simulink model "Semi_Final_integration"  (R2023b)
settings: Solver=FixedStepAuto  StartTime=0.0  StopTime=inf  FixedStep=Ts  RelTol=1e-3
InitFcn:
  | params
  | pin_params
values from neighbouring files (symbols this model uses):
  b = 100    [params.m]
  default1 = 360    [params.m]
  den_Gd = Gd.Den{:}    [params.m]
  encoder_scale = 1/12/4 *2*pi    (= 0.1308996939)    [params.m]
  f = 100    [params.m]
  J = 0.02    [params.m]
  Kb = 0.1    [params.m]
  KD = 0    [params.m]
  Kf = 0.01    [params.m]
  KI = 0.03    [params.m]
  Km = 1    [params.m]
  KP = 0.009    [params.m]
  l = 100    [params.m]
  L = 0.5    [params.m]
  num_Gd = Gd.Num{:}    [params.m]
  r = 100    [params.m]
  R = 2.0    (= 2)    [params.m]
  steering = 0.02    [params.m]
  Vlim = 12    [params.m]
undefined symbols (not defined in the file or in its folder): Wref
libraries: arduinolib x29, arduinosensorlib x17, simulink x6
(part 1 of 2)
settings Model: SimulationMode=external  ExtModeTrigDuration=2  Creator=SJ  LastModifiedBy=SJ
settings SolverCC: AutoInsertRateTranBlk=on
settings OptimizationCC: EnhancedBackFolding=on  PassReuseOutputArgsAs=Individual arguments  ZeroExternalMemoryAtStartup=off  ZeroInternalMemoryAtStartup=off  MaxStackSize=64  OptimizeBlockOrder=speed  DifferentSizesBufferReuse=on  OptimizationCustomize=off  EfficientTunableParamExpr=on
settings DebuggingCC: MultiTaskRateTransMsg=warning  ParameterTunabilityLossMsg=error
settings HardwareCC: ProdBitPerInt=16  ProdBitPerPointer=16  ProdBitPerSizeT=16  ProdBitPerPtrDiffT=16  ProdLargestAtomicFloat=None  ProdWordSize=8  ProdHWDeviceType=Atmel->AVR
settings SFSimCC: MATLABDynamicMemAlloc=off
settings RTWCC: Description=Embedded Coder  SystemTargetFile=ert.tlc  HardwareBoard=Arduino Mega 2560  TemplateMakefile=ert_default_tmf  Toolchain=Arduino AVR  BuildConfiguration=Faster Runs
settings CodeAppCC: ForceParamTrailComments=on  IgnoreCustomStorageClasses=off  OperatorAnnotations=on  SimulinkDataObjDesc=on  SFDataObjDesc=on  InsertBlockDesc=on
settings ERTTargetCC: SupportContinuousTime=on  SupportVariableSizeSignals=on  ExtMode=on  ExtModeTransport=3  ExtModeStaticAlloc=on  ExtModeAutomaticAllocSize=off  ExtModeStaticAllocSize=2048  ExtModeMexFile=ext_xcp  ExtModeMexArgs=0 13 921600  ExtModeIntrfLevel=Level2 - Open

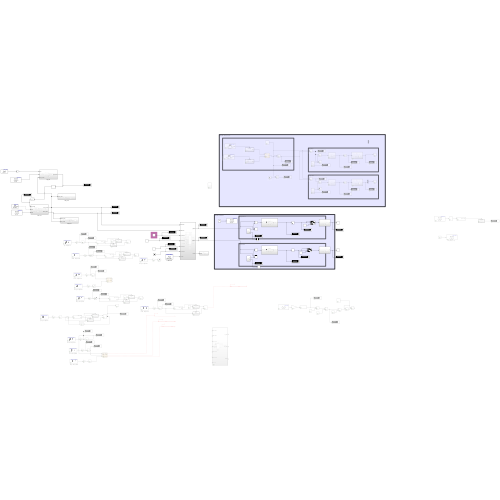
[thumbnail: Simulink's stored preview of the top-level diagram]
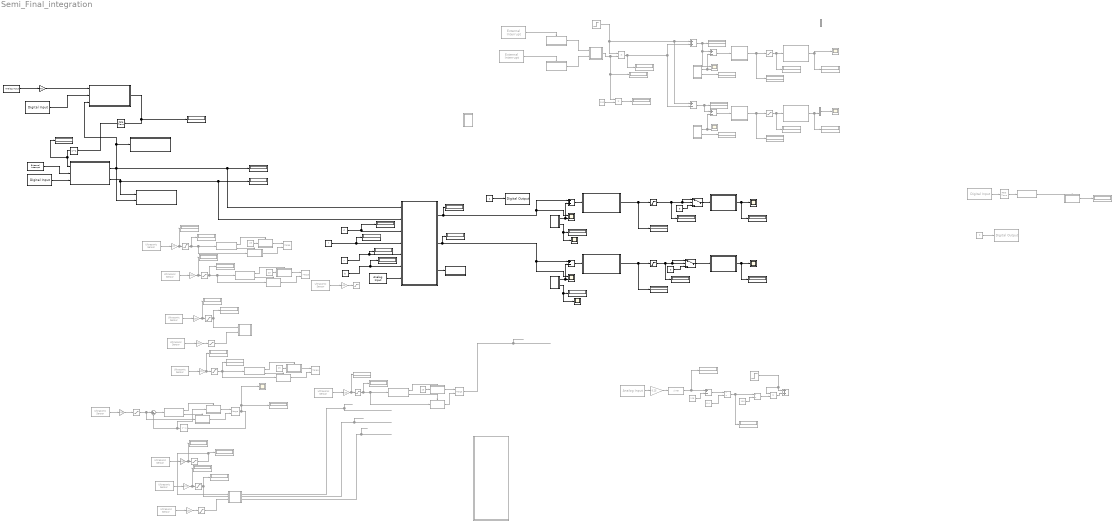
== system Semi_Final_integration ==
  note: Subsystem3
  note: Subsystem13
  note: Left Motor
  note: Variable resistance
  note: sw1,2로 1퍼 증가, 감소
  note: Right Motor
  Add : Sum  Commented=on
  Add{1..2,7..8} (4 alike) : Sum  Commented=on  Inputs=+-
  Add3 : Sum
  Add4 : Sum  Commented=on
  Add5 : Sum  Inputs=+-
  Analog Input : arduinolib/Analog Input  Commented=on  pinNumber=8  ReadResultsOnly=off  ConversionTriggerSource=Software  ExternalTriggerType=uint32( 0 )  OutputDataType=uint16  EnableConversionCompleteNotify=off  EnableOuputStatus=off  SampleTime=-1  blockPlatform=arduino
  Analog Input1 : arduinolib/Analog Input  pinNumber=BS  ReadResultsOnly=off  ConversionTriggerSource=Software  ExternalTriggerType=uint32( 0 )  OutputDataType=uint16  EnableConversionCompleteNotify=off  EnableOuputStatus=off  SampleTime=-1  blockPlatform=arduino
  Chart : Stateflow chart  Commented=on  TreatAsAtomicUnit=on
  Chart1 : Stateflow chart  Commented=on  TreatAsAtomicUnit=on
      settings: PortSchema="{\"entries\":[{\"content\":{\"sides\":[{\"content\":{\"connectorIds\":[\"In1\",\"In2\"]},\"type\":\"ConnectorPlacement.EquallySpacedRectSide\",\"uuid\":\"caf7ae87-23bd-4c3e-9883-bf517c2acc71\"},{\"content\":{\"connectorIds\":[\"Out2\",\"Out1\"],\"side\":\"RIGHT\"},\"type\":\"ConnectorPlacement.EquallySpacedRectSide\",\"uuid\":\"5b72cbb9-a353-4fa8-8bce-0f613714d9b8\"},{\"content\":{\"side\":\"TOP\"},\"type\":\"ConnectorPlacement.EquallySpacedRectSide\",\"uuid\":\"2518c824-60ae-4861-9582-6b6ed29bfb4f\"}]},\"type\":\"ConnectorPlacement.EquallySpacedConnector\",\"uuid\":\"4f310b78-9bfc-4c18-9eab-8f3bf0529cab\"}],\"packageUris\":[\"http://schema.mathworks.com/mf0/Connector/R2020b\"],\"version\":\"1.0\"}"
  Chart2 : Stateflow chart  Commented=on  TreatAsAtomicUnit=on
      settings: PortSchema="{\"entries\":[{\"content\":{\"sides\":[{\"content\":{\"connectorIds\":[\"In1\",\"In2\",\"In3\"]},\"type\":\"ConnectorPlacement.EquallySpacedRectSide\",\"uuid\":\"caf7ae87-23bd-4c3e-9883-bf517c2acc71\"},{\"content\":{\"connectorIds\":[\"Out1\",\"Out3\",\"Out2\"],\"side\":\"RIGHT\"},\"type\":\"ConnectorPlacement.EquallySpacedRectSide\",\"uuid\":\"5b72cbb9-a353-4fa8-8bce-0f613714d9b8\"},{\"content\":{\"side\":\"TOP\"},\"type\":\"ConnectorPlacement.EquallySpacedRectSide\",\"uuid\":\"2518c824-60ae-4861-9582-6b6ed29bfb4f\"}]},\"type\":\"ConnectorPlacement.EquallySpacedConnector\",\"uuid\":\"4f310b78-9bfc-4c18-9eab-8f3bf0529cab\"}],\"packageUris\":[\"http://schema.mathworks.com/mf0/Connector/R2020b\"],\"version\":\"1.0\"}"
  Constant : Constant  Commented=on  Value=128
  Constant1 : Constant  Commented=on  Value=6.4
  Constant{10..12,15} (4 alike) : Constant  Commented=on  Value=25
  Constant13 : Constant
  Constant16 : Constant  Value=0
  Constant2 : Constant  Commented=on  Value=100
  Constant3 : Constant  Commented=on  Value=100
  Constant4 : Constant  Value=f
  Constant5 : Constant  Commented=on  Value=0
  Constant6 : Constant  Value=l
  Constant7 : Constant  Value=b
  Constant8 : Constant  Value=r
  Constant9 : Constant  Value=0
  Data Type Conversion : DataTypeConversion  Commented=on  OutDataTypeStr=uint8  SaturateOnIntegerOverflow=off  RndMeth=Floor
  Delay : Delay  DelayLength=1
  Delay1 : Delay  Commented=on  DelayLength=1
  Digital Input : arduinolib/Digital Input  Commented=on  pinNumber=20  mode=Default  Direction=input  SampleTime=0.1  blockPlatform=arduino
  Digital Input1 : arduinolib/Digital Input  pinNumber=SW3  mode=Default  Direction=input  SampleTime=0.1  blockPlatform=arduino
  Digital Input2 : arduinolib/Digital Input  pinNumber=SW2  mode=Default  Direction=input  SampleTime=0.1  blockPlatform=arduino
  Digital Output : arduinolib/Digital Output  pinNumber=13  Direction=output  blockPlatform=arduino
  Display{,1..7,12,17..23,34..44,47..50} (31 alike) : Display  Commented=on
  Display{8..11,13..16,24..33} (18 alike) : Display
  Divide : Product  Commented=on  Inputs=**
  Divide1 : Product  Commented=on  Inputs=*/
  Divide2 : Product  Commented=on  Inputs=**
  Divide3 : Product  Commented=on  Inputs=*/
  Divide4 : Product  Commented=on  Inputs=**
  External Interrupt : arduinolib/External Interrupt  Commented=on  Pin=20  PullUp=off  Mode=FALLING  InterruptSimulationInput=off
  External Interrupt1 : arduinolib/External Interrupt  Commented=on  Pin=21  PullUp=off  Mode=FALLING  InterruptSimulationInput=off
  External Interrupt2 : arduinolib/External Interrupt  Pin=SW1  PullUp=off  Mode=RISING  InterruptSimulationInput=off
  Function-Call Subsystem1 : Subsystem  Commented=on  TreatAsAtomicUnit=on
  Function-Call Subsystem4 : Subsystem  Commented=on  TreatAsAtomicUnit=on
  Gain : Gain  Commented=on  Gain=0.25
  Gain{1..11} (11 alike) : Gain  Commented=on  Gain=100
  Gain12 : Gain  Gain=70
  If : If  Commented=on  IfExpression=u1 == 0  ShowElse=off
  If Action Subsystem : Subsystem  Commented=on  TreatAsAtomicUnit=on
  If Action Subsystem1 : Subsystem  Commented=on  TreatAsAtomicUnit=on
  If Action Subsystem10 : Subsystem  Commented=on  TreatAsAtomicUnit=on
  If Action Subsystem11 : Subsystem  Commented=on  TreatAsAtomicUnit=on
  If Action Subsystem12 : Subsystem  Commented=on  TreatAsAtomicUnit=on
  If Action Subsystem2 : Subsystem  Commented=on  TreatAsAtomicUnit=on
  If Action Subsystem3 : Subsystem  Commented=on  TreatAsAtomicUnit=on
  If Action Subsystem4 : Subsystem  Commented=on  TreatAsAtomicUnit=on
  If Action Subsystem5 : Subsystem  Commented=on  TreatAsAtomicUnit=on
  If Action Subsystem6 : Subsystem  Commented=on  TreatAsAtomicUnit=on
  If Action Subsystem7 : Subsystem  Commented=on  TreatAsAtomicUnit=on
  If1 : If  Commented=on  IfExpression=u1 > 25
  If2 : If  Commented=on  IfExpression=u1 > 12
  If3 : If  Commented=on  IfExpression=u1 > 25
  If5 : If  Commented=on  IfExpression=u1 > 12
  If6 : If  Commented=on  IfExpression=u1 > 25
  LED_B Ctrl : Subsystem
  LED_R Ctrl : Subsystem
  Merge{1..3,5..6} (5 alike) : Merge  Commented=on
  Mux1 : Mux  Commented=on  Inputs=2
  Mux4 : Mux  Commented=on  Inputs=2
  R_Motor(반시계) : arduinolib/Digital Output  Commented=on  pinNumber=Motor_R_Direction  Direction=output  blockPlatform=arduino
  Rate Transition : RateTransition  Commented=on  OutPortSampleTime=0.5
  Rate Transition1 : RateTransition  Integrity=off
  Saturation : Saturate  Commented=on  UpperLimit=12  LowerLimit=0
  Saturation1 : Saturate  UpperLimit=12  LowerLimit=2
  Saturation{4..6,9..11,13..14} (8 alike) : Saturate  Commented=on  UpperLimit=30  LowerLimit=0
  Saturation12 : Saturate  Commented=on  UpperLimit=15  LowerLimit=0
  Saturation2 : Saturate  UpperLimit=12  LowerLimit=0
  Saturation3 : Saturate  Commented=on  UpperLimit=12  LowerLimit=0
  Saturation7 : Saturate  Commented=on  UpperLimit=15  LowerLimit=0
  Saturation8 : Saturate  Commented=on  UpperLimit=15  LowerLimit=0
  Scope : Scope  Commented=on  NumInputPorts=2
  Scope1 : Scope  NumInputPorts=2
  Scope{2,5,9..10} (4 alike) : Scope
  Scope3 : Scope  Commented=on
  Scope4 : Scope  NumInputPorts=2
  Scope6 : Scope  Commented=on  NumInputPorts=2
  Scope7 : Scope  Commented=on
  Scope8 : Scope  Commented=on
  State_Ctrl : Subsystem
  Step : Step  Commented=on  After=Wref  SampleTime=0
  Step1 : Step  Commented=on  After=Wref  SampleTime=0
  Subsystem : Subsystem  Commented=on
  Subsystem1 : Subsystem  Commented=on
  Subsystem10 : Subsystem  Commented=on
  Subsystem11 : Subsystem  Commented=on
  Subsystem12 : Subsystem  Commented=on
  Subsystem13 : Subsystem
  Subsystem14 : Subsystem
  Subsystem15 : Subsystem
  Subsystem2 : Subsystem  Commented=on
  Subsystem3 : Subsystem
  Subsystem4 : Subsystem
  Subsystem5 : Subsystem  Commented=on
  Subsystem6 : Subsystem  Commented=on
  Subsystem7 : Subsystem
  Subsystem8 : Subsystem
  Subsystem9 : Subsystem
  Sum : Sum  Commented=on  Inputs=|+-
  Switch : Switch  Criteria=u2 > Threshold  Threshold=1.6  SaturateOnIntegerOverflow=off  InputSameDT=off
  Switch1 : Switch  Criteria=u2 > Threshold  Threshold=1.6  SaturateOnIntegerOverflow=off  InputSameDT=off
  light_Ctrl : Subsystem
  가변저항 : arduinolib/Analog Input  pinNumber=8  ReadResultsOnly=off  ConversionTriggerSource=Software  ExternalTriggerType=uint32( 0 )  OutputDataType=uint16  EnableConversionCompleteNotify=off  EnableOuputStatus=off  SampleTime=-1  blockPlatform=arduino
  앞 초음파1 : arduinosensorlib/Ultrasonic Sensor  Commented=on  NumSignalPins=2  TrigPin=F_Triger  EchoPin=F_Echo  SignalPin=3  SampleTime_=0.01  blockPlatform=ARDUINO
  우측 초음파1 : arduinosensorlib/Ultrasonic Sensor  Commented=on  NumSignalPins=2  TrigPin=R_Triger  EchoPin=R_Echo  SignalPin=3  SampleTime_=0.01  blockPlatform=ARDUINO
  우측 초음파2 : arduinosensorlib/Ultrasonic Sensor  Commented=on  NumSignalPins=2  TrigPin=R_Triger  EchoPin=R_Echo  SignalPin=3  SampleTime_=0.01  blockPlatform=ARDUINO
  우측 초음파3 : arduinosensorlib/Ultrasonic Sensor  Commented=on  NumSignalPins=2  TrigPin=R_Triger  EchoPin=R_Echo  SignalPin=3  SampleTime_=0.01  blockPlatform=ARDUINO
  전방 초음파1 : arduinosensorlib/Ultrasonic Sensor  Commented=on  NumSignalPins=2  TrigPin=F_Triger  EchoPin=F_Echo  SignalPin=3  SampleTime_=0.01  blockPlatform=ARDUINO
  좌측 초음파2 : arduinosensorlib/Ultrasonic Sensor  Commented=on  NumSignalPins=2  TrigPin=L_Triger  EchoPin=L_Echo  SignalPin=3  SampleTime_=0.01  blockPlatform=ARDUINO
  좌측 초음파3 : arduinosensorlib/Ultrasonic Sensor  Commented=on  NumSignalPins=2  TrigPin=L_Triger  EchoPin=L_Echo  SignalPin=3  SampleTime_=0.01  blockPlatform=ARDUINO
  후방 초음파{1..4} (4 alike) : arduinosensorlib/Ultrasonic Sensor  Commented=on  NumSignalPins=2  TrigPin=B_Triger  EchoPin=B_Echo  SignalPin=3  SampleTime_=0.01  blockPlatform=ARDUINO
  wires:
  Subsystem/1(Out1) -> Add1/2, Scope/2
  Saturation/1 -> Subsystem1/1(In2), Display/1
  Subsystem1/1(Out1) -> Scope3/1, Display3/1
  External Interrupt/1 -> Function-Call Subsystem4/Trigger
  External Interrupt1/1 -> Function-Call Subsystem1/Trigger
  Function-Call Subsystem4/1(sw1) -> Chart/1(sw1)
  Function-Call Subsystem1/1(sw2) -> Chart/2(sw2)
  Step/1 -> Divide/1, Add8/1, Add/1
  Divide/1 -> Display1/1, Add/2, Add8/2
  Chart/1(n) -> Divide4/1, Display7/1, Divide/2
  Subsystem/2(Out2) -> Display5/1
  Add/1 -> Scope/1, Add1/1, Display4/1
  Subsystem6/1(Out1) -> Display2/1, Saturation/1
  Add1/1 -> Subsystem6/1(In1)
  Add7/1 -> Subsystem12/1(In1)
  Subsystem11/1(Out1) -> Display19/1, Mux4/2
  Saturation3/1 -> Subsystem11/1(In2), Display17/1
  Mux4/1 -> Scope7/1
  Subsystem10/1(Out1) -> Add7/2, Scope6/2
  Subsystem12/1(Out1) -> Display18/1, Saturation3/1
  Subsystem10/2(Out2) -> Display20/1
  Add8/1 -> Add7/1, Display21/1
  Divide4/1 -> Display22/1
  Constant3/1 -> Divide4/2
  Digital Input/1 -> Rate Transition/1
  If/1 -> If Action Subsystem/Action
  If Action Subsystem/1(Out1) -> Display23/1
  Rate Transition/1 -> If/1
  Constant5/1 -> R_Motor(반시계)/1
  Digital Input1/1 -> light_Ctrl/2(In2)
  light_Ctrl/1(light_mode) -> Display10/1, Rate Transition1/1
  Analog Input1/1 -> Gain12/1
  Rate Transition1/1 -> Delay/1
  External Interrupt2/1 -> State_Ctrl/2(SW1)
  Delay/1 -> Display11/1, State_Ctrl/1(light_mode)
  Digital Input2/1 -> State_Ctrl/3(SW2)
  Add2/1 -> Divide1/1
  Data Type Conversion/1 -> Display12/1, Add2/1
  Gain/1 -> Data Type Conversion/1
  Constant/1 -> Add2/2
  Constant2/1 -> Divide3/2
  Step1/1 -> Add4/1, Divide2/1
  Divide3/1 -> Divide2/2
  Constant1/1 -> Divide1/2
  Analog Input/1 -> Gain/1
  Divide2/1 -> Add4/2
  Divide1/1 -> Display6/1, Divide3/1
  가변저항/1 -> Subsystem4/7(가변저항)
  Subsystem4/1(L_Motor) -> Add3/1, Scope1/1, Display24/1
  Subsystem8/1(Out1) -> Scope2/1, Display26/1
  Subsystem7/1(Out1) -> Add3/2, Scope1/2
  Subsystem9/1(Out1) -> Display29/1, Saturation1/1
  Subsystem7/2(Out2) -> Scope10/1, Display27/1
  Add3/1 -> Subsystem9/1(In1)
  Subsystem4/2(R_Motor) -> Scope4/1, Add5/1, Display25/1
  Subsystem14/1(Out1) -> Scope5/1, Display30/1
  Subsystem13/1(Out1) -> Add5/2, Scope4/2
  Subsystem15/1(Out1) -> Display33/1, Saturation2/1
  Subsystem13/2(Out2) -> Scope9/1, Display31/1
  Add5/1 -> Subsystem15/1(In1)
  우측 초음파2/1 -> Gain3/1
  Gain3/1 -> Display35/1, Saturation4/1
  Saturation4/1 -> Chart1/1(RUS), Display34/1
  Delay1/1 -> If Action Subsystem6/1(In1), Sum/2
  전방 초음파1/1 -> Gain2/1
  Sum/1 -> If3/1
  Merge3/1 -> Scope8/1, Display36/1, Delay1/1
  If Action Subsystem7/1(전방 초음파) -> Merge3/2
  If3/2 -> If Action Subsystem7/Action
  Gain2/1 -> Saturation5/1
  Saturation5/1 -> If Action Subsystem7/1(In1), Sum/1
  If Action Subsystem6/1(Out1) -> Merge3/1
  If3/1 -> If Action Subsystem6/Action
  Constant10/1 -> If Action Subsystem1/1(In1)
  If Action Subsystem2/1(전방 초음파) -> Merge1/2
  Saturation6/1 -> If1/1, Display37/1, If Action Subsystem2/1(In1)
  If1/2 -> If Action Subsystem2/Action
  Gain1/1 -> Display38/1, Saturation6/1
  If1/1 -> If Action Subsystem1/Action
  후방 초음파1/1 -> Gain1/1
  If Action Subsystem1/1(Out1) -> Merge1/1
  좌측 초음파2/1 -> Gain4/1
  If Action Subsystem3/1(Out1) -> Merge2/1
  If2/1 -> If Action Subsystem3/Action
  Gain4/1 -> Display40/1, Saturation7/1
  If2/2 -> If Action Subsystem4/Action
  If Action Subsystem4/1(전방 초음파) -> Merge2/2
  Constant11/1 -> If Action Subsystem3/1(In1)
  Saturation7/1 -> Display39/1, If2/1, If Action Subsystem4/1(In1)
  Saturation8/1 -> Display41/1, If5/1, If Action Subsystem10/1(In1)
  If5/1 -> If Action Subsystem5/Action
  앞 초음파1/1 -> Gain5/1
  If5/2 -> If Action Subsystem10/Action
  If Action Subsystem10/1(전방 초음파) -> Merge5/2
  If Action Subsystem5/1(Out1) -> Merge5/1
  Constant12/1 -> If Action Subsystem5/1(In1)
  Gain5/1 -> Display42/1, Saturation8/1
  State_Ctrl/1(Drive_mode) -> Subsystem4/1(drive mode), Display8/1, light_Ctrl/3(Drive_mode1), LED_R Ctrl/1(Drive_mode), LED_B Ctrl/2(Drive_mode)
  Constant4/1 -> Display16/1, Subsystem4/3(전방 초음파)
  Gain6/1 -> Saturation9/1
  후방 초음파2/1 -> Gain6/1
  Merge6/1 -> ?
  Constant15/1 -> If Action Subsystem11/1(In1)
  If Action Subsystem12/1(전방 초음파) -> Merge6/2
  Saturation10/1 -> Display43/1, If6/1, If Action Subsystem12/1(In1)
  If6/2 -> If Action Subsystem12/Action
  Gain7/1 -> Display44/1, Saturation10/1
  If6/1 -> If Action Subsystem11/Action
  우측 초음파1/1 -> Gain7/1
  If Action Subsystem11/1(Out1) -> Merge6/1
  Saturation9/1 -> Chart1/2(BUS)
  Gain11/1 -> Display50/1, Saturation12/1
  Gain10/1 -> Saturation14/1
  Chart2/2(data3) -> ?
  후방 초음파3/1 -> Gain10/1
  Chart2/1(data1) -> ?
  좌측 초음파3/1 -> Gain11/1
  Chart2/3(data2) -> ?
  Saturation14/1 -> Chart2/3(BUS)
  Gain9/1 -> Display48/1, Saturation13/1
  Saturation12/1 -> Display49/1, Chart2/1(LUS)
  Saturation13/1 -> Chart2/2(RUS), Display47/1
  우측 초음파3/1 -> Gain9/1
  Constant6/1 -> Display15/1, Subsystem4/4(좌측 초음파)
  Constant8/1 -> Display14/1, Subsystem4/5(우측 초음파)
  Gain8/1 -> Saturation11/1
  후방 초음파4/1 -> Gain8/1
  Subsystem4/3(buzzer) -> Subsystem3/1(buzzer)
  Constant7/1 -> Display13/1, Subsystem4/6(후방 초음파)
  Gain12/1 -> light_Ctrl/1(light1)
  Constant13/1 -> Digital Output/1
  State_Ctrl/2(ADAS_state1) -> LED_B Ctrl/1(ADAS_state), Subsystem4/2(adas mode), Display9/1
  Constant9/1 -> Switch/3
  Saturation2/1 -> Display28/1, Switch/1, Switch/2
  Switch/1 -> Subsystem14/1(In2)
  Saturation1/1 -> Switch1/1, Switch1/2, Display32/1
  Constant16/1 -> Switch1/3
  Switch1/1 -> Subsystem8/1(In2)

== system Semi_Final_integration/Function-Call Subsystem1 ==
  function : TriggerPort  TriggerType=function-call  VariantControl=(inherit)
  Add : Sum  Inputs=+-
  Constant : Constant
  Delay : Delay  DelayLength=1
  sw2 : Outport
  wires:
  Add/1 -> Delay/1, sw2/1
  Delay/1 -> Add/2
  Constant/1 -> Add/1

== system Semi_Final_integration/Function-Call Subsystem4 ==
  function : TriggerPort  TriggerType=function-call  VariantControl=(inherit)
  Add : Sum  Inputs=+-
  Constant : Constant
  Delay : Delay  DelayLength=1
  sw1 : Outport
  wires:
  Add/1 -> sw1/1, Delay/1
  Delay/1 -> Add/2
  Constant/1 -> Add/1

== system Semi_Final_integration/If Action Subsystem ==
  Action Port : ActionPort  ActionPortLabel=if(u1 == 0)
  Add : Sum
  Constant : Constant
  Constant1 : Constant  Value=3
  Delay : Delay  DelayLength=1
  Mod : Math  Operator=mod
  Out1 : Outport
  wires:
  Mod/1 -> Delay/1, Out1/1
  Delay/1 -> Add/2
  Constant/1 -> Add/1
  Add/1 -> Mod/1
  Constant1/1 -> Mod/2

== system Semi_Final_integration/If Action Subsystem1 ==
  In1 : Inport
  Action Port : ActionPort  ActionPortLabel=if(u1 > 25)
  Out1 : Outport
  wires:
  In1/1 -> Out1/1

== system Semi_Final_integration/If Action Subsystem10 ==
  In1 : Inport
  Action Port : ActionPort  ActionPortLabel=else
  전방 초음파 : Outport
  wires:
  In1/1 -> 전방 초음파/1

== system Semi_Final_integration/If Action Subsystem11 ==
  In1 : Inport
  Action Port : ActionPort  ActionPortLabel=if(u1 > 25)
  Out1 : Outport
  wires:
  In1/1 -> Out1/1

== system Semi_Final_integration/If Action Subsystem12 ==
  In1 : Inport
  Action Port : ActionPort  ActionPortLabel=else
  전방 초음파 : Outport
  wires:
  In1/1 -> 전방 초음파/1

== system Semi_Final_integration/If Action Subsystem2 ==
  In1 : Inport
  Action Port : ActionPort  ActionPortLabel=else
  전방 초음파 : Outport
  wires:
  In1/1 -> 전방 초음파/1

== system Semi_Final_integration/If Action Subsystem3 ==
  In1 : Inport
  Action Port : ActionPort  ActionPortLabel=if(u1 > 12)
  Out1 : Outport
  wires:
  In1/1 -> Out1/1

== system Semi_Final_integration/If Action Subsystem4 ==
  In1 : Inport
  Action Port : ActionPort  ActionPortLabel=else
  전방 초음파 : Outport
  wires:
  In1/1 -> 전방 초음파/1

== system Semi_Final_integration/If Action Subsystem5 ==
  In1 : Inport
  Action Port : ActionPort  ActionPortLabel=if(u1 > 12)
  Out1 : Outport
  wires:
  In1/1 -> Out1/1

== system Semi_Final_integration/If Action Subsystem6 ==
  In1 : Inport
  Action Port : ActionPort  ActionPortLabel=if(u1 > 25)
  Out1 : Outport
  wires:
  In1/1 -> Out1/1

== system Semi_Final_integration/If Action Subsystem7 ==
  In1 : Inport
  Action Port : ActionPort  ActionPortLabel=else
  전방 초음파 : Outport
  wires:
  In1/1 -> 전방 초음파/1

== system Semi_Final_integration/LED_B Ctrl ==
  ADAS_state : Inport
  Drive_mode : Inport  Port=2
  Constant : Constant
  Digital Output : arduinolib/Digital Output  pinNumber=LED1_B  Direction=output  blockPlatform=arduino
  If Action Subsystem1 : Subsystem  TreatAsAtomicUnit=on
  If Action Subsystem3 : Subsystem  TreatAsAtomicUnit=on
  If1 : If  IfExpression=u1 ==1
  Merge : Merge
  Product : Product
  Product1 : Product
  Pulse Generator : DiscretePulseGenerator  PulseType=Time based  PulseWidth=50
  wires:
  If1/2 -> If Action Subsystem3/Action
  If Action Subsystem1/1(Out1) -> Merge/1
  ADAS_state/1 -> If1/1
  If1/1 -> If Action Subsystem1/Action
  Merge/1 -> Digital Output/1
  If Action Subsystem3/1(Out1) -> Merge/2
  Drive_mode/1 -> Product/1, Product1/2
  Pulse Generator/1 -> Product/2
  Constant/1 -> Product1/1
  Product1/1 -> If Action Subsystem1/1(Input)
  Product/1 -> If Action Subsystem3/1(Input)

== system Semi_Final_integration/LED_R Ctrl ==
  Drive_mode : Inport
  Digital Output : arduinolib/Digital Output  pinNumber=LED1_R  Direction=output  blockPlatform=arduino
  If Action Subsystem1 : Subsystem  TreatAsAtomicUnit=on
  If Action Subsystem3 : Subsystem  TreatAsAtomicUnit=on
  If1 : If  IfExpression=u1 ==1
  Merge : Merge
  wires:
  If1/2 -> If Action Subsystem3/Action
  If Action Subsystem1/1(Out1) -> Merge/1
  Drive_mode/1 -> If1/1
  If1/1 -> If Action Subsystem1/Action
  Merge/1 -> Digital Output/1
  If Action Subsystem3/1(Out1) -> Merge/2

== system Semi_Final_integration/State_Ctrl ==
  light_mode : Inport
  SW1 : Inport  Port=2
  SW2 : Inport  Port=3
  ADAS_state : Subsystem
  Delay : Delay  DelayLength=1
  If : If  IfExpression=u1 ==1  ShowElse=off
  Rate Transition2 : RateTransition  Integrity=off  OutPortSampleTime=0.01
  drive_mode : Subsystem
  Drive_mode : Outport
  ADAS_state1 : Outport  Port=2
  wires:
  If/1 -> ADAS_state/1(In1)
  drive_mode/1(D_mode) -> If/1, Drive_mode/1
  ADAS_state/1(ADAS_state) -> Delay/1, ADAS_state1/1
  SW1/1 -> drive_mode/2(sw1)
  Delay/1 -> drive_mode/3(A_state)
  light_mode/1 -> drive_mode/1(light_mode)
  SW2/1 -> Rate Transition2/1
  Rate Transition2/1 -> ADAS_state/2(In2)

== system Semi_Final_integration/Subsystem ==
  Data Type Conversion1 : DataTypeConversion  OutDataTypeStr=int32  SaturateOnIntegerOverflow=off  RndMeth=Floor
  Discrete Transfer Fcn : DiscreteTransferFcn  Numerator=num_Gd  Denominator=den_Gd
  Discrete Derivative : simulink/Discrete/Discrete Derivative  gainval=1.0  ICPrevScaledInput=0.0  OutMin=[]  OutMax=[]  OutDataType=fixdt(1, 16)  OutScaling=2^-10  DoSatur=off
  Display : Display
  Encoder : arduinosensorlib/Encoder  InputA=18  InputB=19  Mode=No reset  SampleTime=-1
  Gain1 : Gain  Gain=encoder_scale
  Gain2 : Gain  Gain=60/(2*pi)
  Out1 : Outport
  Out2 : Outport  Port=2
  wires:
  Gain1/1 -> Display/1, Gain2/1, Data Type Conversion1/1
  Encoder/1 -> Discrete Derivative/1
  Gain2/1 -> Out2/1
  Data Type Conversion1/1 -> Discrete Transfer Fcn/1
  Discrete Derivative/1 -> Gain1/1
  Discrete Transfer Fcn/1 -> Out1/1

== system Semi_Final_integration/Subsystem1 ==
  In2 : Inport
  Add : Sum  Commented=on  Inputs=+-
  Add1 : Sum  Commented=on
  Data Type Conversion : DataTypeConversion  OutDataTypeStr=uint8  SaturateOnIntegerOverflow=off  RndMeth=Floor
  Data Type Conversion1 : DataTypeConversion  OutDataTypeStr=double  SaturateOnIntegerOverflow=off  RndMeth=Floor
  Display1 : Display
  Gain : Gain  Commented=on  Gain=Kb
  Gain1 : Gain  Gain=255/Vlim
  PWM : arduinolib/PWM  pinNumber=11  frequencyType=Default  desiredFrequency=490.2  achievableFrequency=490.2
  Transfer Fcn : TransferFcn  Commented=on  Numerator=Km  Denominator=[L R]
  Transfer Fcn1 : TransferFcn  Commented=on  Numerator=1  Denominator=[J Kf]
  Out1 : Outport
  wires:
  ? -> Add/1
  ? -> Add1/1
  Add/1 -> Transfer Fcn/1
  Add1/1 -> Transfer Fcn1/1
  Transfer Fcn/1 -> Add1/2
  Gain/1 -> Add/2
  Transfer Fcn1/1 -> Gain/1
  In2/1 -> Gain1/1
  Gain1/1 -> Data Type Conversion/1
  Data Type Conversion1/1 -> Out1/1
  Data Type Conversion/1 -> Data Type Conversion1/1, Display1/1, PWM/1

== system Semi_Final_integration/Subsystem10 ==
  Data Type Conversion1 : DataTypeConversion  OutDataTypeStr=int32  SaturateOnIntegerOverflow=off  RndMeth=Floor
  Discrete Transfer Fcn : DiscreteTransferFcn  Numerator=num_Gd  Denominator=den_Gd
  Discrete Derivative : simulink/Discrete/Discrete Derivative  gainval=1.0  ICPrevScaledInput=0.0  OutMin=[]  OutMax=[]  OutDataType=fixdt(1, 16)  OutScaling=2^-10  DoSatur=off
  Display : Display
  Encoder : arduinosensorlib/Encoder  InputA=20  InputB=21  Mode=No reset  SampleTime=-1
  Gain1 : Gain  Gain=encoder_scale
  Gain2 : Gain  Gain=60/(2*pi)
  Out1 : Outport
  Out2 : Outport  Port=2
  wires:
  Gain1/1 -> Display/1, Gain2/1, Data Type Conversion1/1
  Encoder/1 -> Discrete Derivative/1
  Gain2/1 -> Out2/1
  Data Type Conversion1/1 -> Discrete Transfer Fcn/1
  Discrete Derivative/1 -> Gain1/1
  Discrete Transfer Fcn/1 -> Out1/1

== system Semi_Final_integration/Subsystem11 ==
  In2 : Inport
  Add : Sum  Commented=on  Inputs=+-
  Add1 : Sum  Commented=on
  Data Type Conversion : DataTypeConversion  OutDataTypeStr=uint8  SaturateOnIntegerOverflow=off  RndMeth=Floor
  Data Type Conversion1 : DataTypeConversion  OutDataTypeStr=double  SaturateOnIntegerOverflow=off  RndMeth=Floor
  Display1 : Display
  Gain : Gain  Commented=on  Gain=Kb
  Gain1 : Gain  Gain=255/Vlim
  PWM : arduinolib/PWM  pinNumber=11  frequencyType=Default  desiredFrequency=490.2  achievableFrequency=490.2
  Transfer Fcn : TransferFcn  Commented=on  Numerator=Km  Denominator=[L R]
  Transfer Fcn1 : TransferFcn  Commented=on  Numerator=1  Denominator=[J Kf]
  Out1 : Outport
  wires:
  ? -> Add/1
  ? -> Add1/1
  Add/1 -> Transfer Fcn/1
  Add1/1 -> Transfer Fcn1/1
  Transfer Fcn/1 -> Add1/2
  Gain/1 -> Add/2
  Transfer Fcn1/1 -> Gain/1
  In2/1 -> Gain1/1
  Gain1/1 -> Data Type Conversion/1
  Data Type Conversion1/1 -> Out1/1
  Data Type Conversion/1 -> Data Type Conversion1/1, Display1/1, PWM/1

== system Semi_Final_integration/Subsystem12 ==
  In1 : Inport
  Derivative1 : Derivative  Commented=on
  Gain4 : Gain  Commented=on  Gain=KI
  Gain5 : Gain  Commented=on  Gain=KP
  Gain6 : Gain  Commented=on  Gain=KD
  Integrator1 : Integrator  Commented=on
  Subtract1 : Sum  Commented=on  Inputs=+++
  Out1 : Outport
  wires:
  Derivative1/1 -> Subtract1/3
  Gain4/1 -> Integrator1/1
  Integrator1/1 -> Subtract1/1
  Gain6/1 -> Derivative1/1
  Subtract1/1 -> Out1/1
  In1/1 -> Gain5/1, Gain6/1, Gain4/1
  Gain5/1 -> Subtract1/2

== system Semi_Final_integration/Subsystem13 ==
  Data Type Conversion1 : DataTypeConversion  OutDataTypeStr=int32  SaturateOnIntegerOverflow=off  RndMeth=Floor
  Discrete Transfer Fcn : DiscreteTransferFcn  Numerator=num_Gd  Denominator=den_Gd
  Discrete Derivative : simulink/Discrete/Discrete Derivative  gainval=1.0  ICPrevScaledInput=0.0  OutMin=[]  OutMax=[]  OutDataType=fixdt(1, 16)  OutScaling=2^-10  DoSatur=off
  Display : Display
  Encoder : arduinosensorlib/Encoder  InputA=20  InputB=21  Mode=No reset  SampleTime=0.01
  Gain1 : Gain  Gain=encoder_scale
  Gain2 : Gain  Gain=60/(2*pi)
  Out1 : Outport
  Out2 : Outport  Port=2
  wires:
  Gain1/1 -> Display/1, Gain2/1, Data Type Conversion1/1
  Encoder/1 -> Discrete Derivative/1
  Gain2/1 -> Out2/1
  Data Type Conversion1/1 -> Discrete Transfer Fcn/1
  Discrete Derivative/1 -> Gain1/1
  Discrete Transfer Fcn/1 -> Out1/1

== system Semi_Final_integration/Subsystem14 ==
  In2 : Inport
  Add : Sum  Commented=on  Inputs=+-
  Add1 : Sum  Commented=on
  Data Type Conversion : DataTypeConversion  OutDataTypeStr=uint8  SaturateOnIntegerOverflow=off  RndMeth=Floor
  Data Type Conversion1 : DataTypeConversion  OutDataTypeStr=double  SaturateOnIntegerOverflow=off  RndMeth=Floor
  Display1 : Display
  Gain : Gain  Commented=on  Gain=Kb
  Gain1 : Gain  Gain=255/Vlim
  PWM : arduinolib/PWM  pinNumber=3  frequencyType=Default  desiredFrequency=490.2  achievableFrequency=490.2
  Transfer Fcn : TransferFcn  Commented=on  Numerator=Km  Denominator=[L R]
  Transfer Fcn1 : TransferFcn  Commented=on  Numerator=1  Denominator=[J Kf]
  Out1 : Outport
  wires:
  ? -> Add/1
  ? -> Add1/1
  Add/1 -> Transfer Fcn/1
  Add1/1 -> Transfer Fcn1/1
  Transfer Fcn/1 -> Add1/2
  Gain/1 -> Add/2
  Transfer Fcn1/1 -> Gain/1
  In2/1 -> Gain1/1
  Gain1/1 -> Data Type Conversion/1
  Data Type Conversion1/1 -> Out1/1
  Data Type Conversion/1 -> Data Type Conversion1/1, Display1/1, PWM/1

== system Semi_Final_integration/Subsystem15 ==
  In1 : Inport
  Derivative2 : Derivative
  Gain1 : Gain  Gain=KI
  Gain2 : Gain  Gain=KP
  Gain3 : Gain  Gain=KD
  Integrator2 : Integrator
  Subtract2 : Sum  Inputs=+++
  Out1 : Outport
  wires:
  Gain1/1 -> Integrator2/1
  Gain2/1 -> Subtract2/2
  Integrator2/1 -> Subtract2/1
  In1/1 -> Gain2/1, Gain3/1, Gain1/1
  Derivative2/1 -> Subtract2/3
  Gain3/1 -> Derivative2/1
  Subtract2/1 -> Out1/1

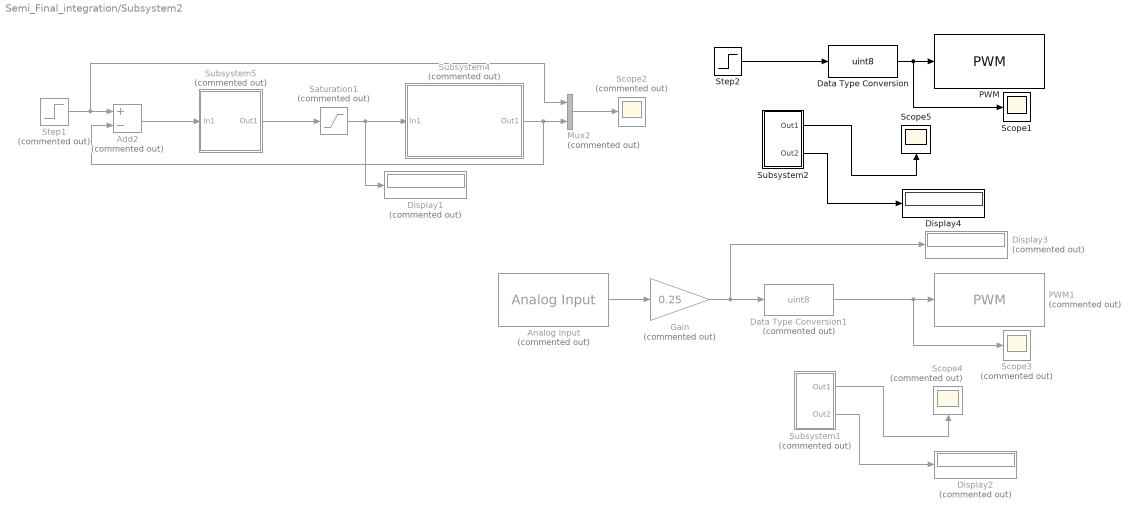
== system Semi_Final_integration/Subsystem2 ==
  Add2 : Sum  Commented=on  Inputs=+-
  Analog Input : arduinolib/Analog Input  Commented=on  pinNumber=8  ReadResultsOnly=off  ConversionTriggerSource=Software  ExternalTriggerType=uint32( 0 )  OutputDataType=uint16  EnableConversionCompleteNotify=off  EnableOuputStatus=off  SampleTime=-1  blockPlatform=arduino
  Data Type Conversion : DataTypeConversion  OutDataTypeStr=uint8  SaturateOnIntegerOverflow=off  RndMeth=Floor
  Data Type Conversion1 : DataTypeConversion  Commented=on  OutDataTypeStr=uint8  SaturateOnIntegerOverflow=off  RndMeth=Floor
  Display1 : Display  Commented=on
  Display2 : Display  Commented=on
  Display3 : Display  Commented=on
  Display4 : Display
  Gain : Gain  Commented=on  Gain=0.25
  Mux2 : Mux  Commented=on  Inputs=2
  PWM : arduinolib/PWM  pinNumber=11  frequencyType=Default  desiredFrequency=490.2  achievableFrequency=490.2
  PWM1 : arduinolib/PWM  Commented=on  pinNumber=11  frequencyType=Default  desiredFrequency=490.2  achievableFrequency=490.2
  Saturation1 : Saturate  Commented=on  UpperLimit=Vlim  LowerLimit=0
  Scope1 : Scope
  Scope2 : Scope  Commented=on
  Scope3 : Scope  Commented=on
  Scope4 : Scope  Commented=on
  Scope5 : Scope
  Step1 : Step  Commented=on  After=Wref  SampleTime=0
  Step2 : Step  After=Wref  SampleTime=0
  Subsystem1 : Subsystem  Commented=on
  Subsystem2 : Subsystem
  Subsystem4 : Subsystem  Commented=on
  Subsystem5 : Subsystem  Commented=on
  wires:
  Data Type Conversion/1 -> Scope1/1, PWM/1
  Add2/1 -> Subsystem5/1(In1)
  Saturation1/1 -> Subsystem4/1(In1), Display1/1
  Mux2/1 -> Scope2/1
  Subsystem4/1(Out1) -> Add2/2, Mux2/2
  Step2/1 -> Data Type Conversion/1
  Subsystem5/1(Out1) -> Saturation1/1
  Step1/1 -> Mux2/1, Add2/1
  Subsystem1/1(Out1) -> Scope4/1
  Gain/1 -> Display3/1, Data Type Conversion1/1
  Data Type Conversion1/1 -> Scope3/1, PWM1/1
  Analog Input/1 -> Gain/1
  Subsystem1/2(Out2) -> Display2/1
  Subsystem2/1(Out1) -> Scope5/1
  Subsystem2/2(Out2) -> Display4/1

== system Semi_Final_integration/Subsystem3 ==
  buzzer : Inport
  If : If  IfExpression=u1 == 1
  If Action Subsystem : Subsystem  TreatAsAtomicUnit=on
  If Action Subsystem1 : Subsystem  TreatAsAtomicUnit=on
  Merge : Merge
  PWM : arduinolib/PWM  pinNumber=9  frequencyType=Default  desiredFrequency=490.2  achievableFrequency=490.2
  wires:
  buzzer/1 -> If/1
  If/1 -> If Action Subsystem/Action
  If/2 -> If Action Subsystem1/Action
  If Action Subsystem/1(Output) -> Merge/1
  If Action Subsystem1/1(Out1) -> Merge/2
  Merge/1 -> PWM/1

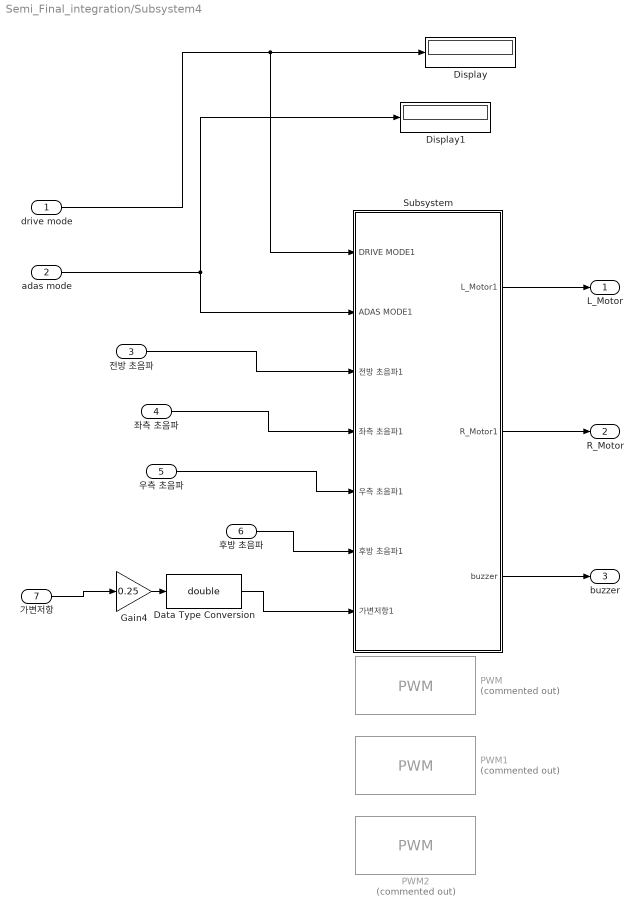
== system Semi_Final_integration/Subsystem4 ==
  drive mode : Inport
  adas mode : Inport  Port=2
  전방 초음파 : Inport  Port=3
  좌측 초음파 : Inport  Port=4
  우측 초음파 : Inport  Port=5
  후방 초음파 : Inport  Port=6
  가변저항 : Inport  Port=7
  Data Type Conversion : DataTypeConversion  OutDataTypeStr=double  SaturateOnIntegerOverflow=off  RndMeth=Floor
  Display : Display
  Display1 : Display
  Gain4 : Gain  Gain=0.25
  PWM : arduinolib/PWM  Commented=on  pinNumber=RGB_LED_1  frequencyType=Default  desiredFrequency=490.2  achievableFrequency=490.2
  PWM1 : arduinolib/PWM  Commented=on  pinNumber=RGB_LED_2  frequencyType=Default  desiredFrequency=490.2  achievableFrequency=490.2
  PWM2 : arduinolib/PWM  Commented=on  pinNumber=RGB_LED_3  frequencyType=Default  desiredFrequency=490.2  achievableFrequency=490.2
  Subsystem : Subsystem
  L_Motor : Outport
  R_Motor : Outport  Port=2
  buzzer : Outport  Port=3
  wires:
  drive mode/1 -> Subsystem/1(DRIVE MODE1), Display/1
  adas mode/1 -> Display1/1, Subsystem/2(ADAS MODE1)
  Subsystem/3(buzzer) -> buzzer/1
  가변저항/1 -> Gain4/1
  Gain4/1 -> Data Type Conversion/1
  Data Type Conversion/1 -> Subsystem/7(가변저항1)
  Subsystem/2(R_Motor1) -> R_Motor/1
  Subsystem/1(L_Motor1) -> L_Motor/1
  전방 초음파/1 -> Subsystem/3(전방 초음파1)
  좌측 초음파/1 -> Subsystem/4(좌측 초음파1)
  우측 초음파/1 -> Subsystem/5(우측 초음파1)
  후방 초음파/1 -> Subsystem/6(후방 초음파1)

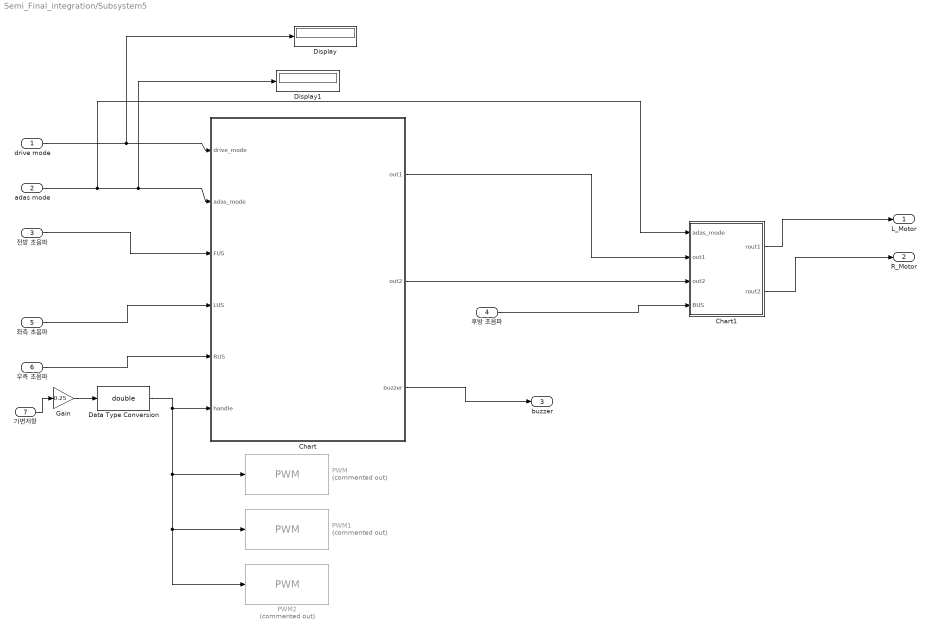
== system Semi_Final_integration/Subsystem5 ==
  drive mode : Inport
  adas mode : Inport  Port=2
  전방 초음파 : Inport  Port=3
  후방 초음파 : Inport  Port=4
  좌측 초음파 : Inport  Port=5
  우측 초음파 : Inport  Port=6
  가변저항 : Inport  Port=7
  Chart : Stateflow chart  TreatAsAtomicUnit=on
  Chart1 : Stateflow chart  TreatAsAtomicUnit=on
  Data Type Conversion : DataTypeConversion  OutDataTypeStr=double  SaturateOnIntegerOverflow=off  RndMeth=Floor
  Display : Display
  Display1 : Display
  Gain : Gain  Gain=0.25
  PWM : arduinolib/PWM  Commented=on  pinNumber=RGB_LED_1  frequencyType=Default  desiredFrequency=490.2  achievableFrequency=490.2
  PWM1 : arduinolib/PWM  Commented=on  pinNumber=RGB_LED_2  frequencyType=Default  desiredFrequency=490.2  achievableFrequency=490.2
  PWM2 : arduinolib/PWM  Commented=on  pinNumber=RGB_LED_3  frequencyType=Default  desiredFrequency=490.2  achievableFrequency=490.2
  L_Motor : Outport
  R_Motor : Outport  Port=2
  buzzer : Outport  Port=3
  wires:
  drive mode/1 -> Chart/1(drive_mode), Display/1
  adas mode/1 -> Chart1/1(adas_mode), Chart/2(adas_mode), Display1/1
  전방 초음파/1 -> Chart/3(FUS)
  후방 초음파/1 -> Chart1/4(BUS)
  좌측 초음파/1 -> Chart/4(LUS)
  우측 초음파/1 -> Chart/5(RUS)
  Chart/3(buzzer) -> buzzer/1
  Chart/1(out1) -> Chart1/2(out1)
  Chart/2(out2) -> Chart1/3(out2)
  Chart1/1(rout1) -> L_Motor/1
  Chart1/2(rout2) -> R_Motor/1
  가변저항/1 -> Gain/1
  Gain/1 -> Data Type Conversion/1
  Data Type Conversion/1 -> PWM2/1, PWM1/1, PWM/1, Chart/6(handle)

== system Semi_Final_integration/Subsystem6 ==
  In1 : Inport
  Derivative1 : Derivative
  Gain4 : Gain  Gain=KI
  Gain5 : Gain  Gain=KP
  Gain6 : Gain  Gain=KD
  Integrator1 : Integrator
  Subtract1 : Sum  Inputs=+++
  Out1 : Outport
  wires:
  Derivative1/1 -> Subtract1/3
  Gain4/1 -> Integrator1/1
  Integrator1/1 -> Subtract1/1
  Gain6/1 -> Derivative1/1
  Subtract1/1 -> Out1/1
  In1/1 -> Gain5/1, Gain6/1, Gain4/1
  Gain5/1 -> Subtract1/2

== system Semi_Final_integration/Subsystem7 ==
  Data Type Conversion1 : DataTypeConversion  OutDataTypeStr=int32  SaturateOnIntegerOverflow=off  RndMeth=Floor
  Discrete Transfer Fcn : DiscreteTransferFcn  Numerator=num_Gd  Denominator=den_Gd
  Discrete Derivative : simulink/Discrete/Discrete Derivative  gainval=1.0  ICPrevScaledInput=0.0  OutMin=[]  OutMax=[]  OutDataType=fixdt(1, 16)  OutScaling=2^-10  DoSatur=off
  Display : Display
  Encoder : arduinosensorlib/Encoder  InputA=18  InputB=19  Mode=No reset  SampleTime=0.01
  Gain1 : Gain  Gain=encoder_scale
  Gain2 : Gain  Gain=60/(2*pi)
  Out1 : Outport
  Out2 : Outport  Port=2
  wires:
  Gain1/1 -> Display/1, Gain2/1, Data Type Conversion1/1
  Encoder/1 -> Discrete Derivative/1
  Gain2/1 -> Out2/1
  Data Type Conversion1/1 -> Discrete Transfer Fcn/1
  Discrete Derivative/1 -> Gain1/1
  Discrete Transfer Fcn/1 -> Out1/1

== system Semi_Final_integration/Subsystem8 ==
  In2 : Inport
  Add : Sum  Commented=on  Inputs=+-
  Add1 : Sum  Commented=on
  Data Type Conversion : DataTypeConversion  OutDataTypeStr=uint8  SaturateOnIntegerOverflow=off  RndMeth=Floor
  Data Type Conversion1 : DataTypeConversion  OutDataTypeStr=double  SaturateOnIntegerOverflow=off  RndMeth=Floor
  Display1 : Display
  Gain : Gain  Commented=on  Gain=Kb
  Gain1 : Gain  Gain=255/Vlim
  PWM : arduinolib/PWM  pinNumber=11  frequencyType=Default  desiredFrequency=490.2  achievableFrequency=490.2
  Transfer Fcn : TransferFcn  Commented=on  Numerator=Km  Denominator=[L R]
  Transfer Fcn1 : TransferFcn  Commented=on  Numerator=1  Denominator=[J Kf]
  Out1 : Outport
  wires:
  ? -> Add/1
  ? -> Add1/1
  Add/1 -> Transfer Fcn/1
  Add1/1 -> Transfer Fcn1/1
  Transfer Fcn/1 -> Add1/2
  Gain/1 -> Add/2
  Transfer Fcn1/1 -> Gain/1
  In2/1 -> Gain1/1
  Gain1/1 -> Data Type Conversion/1
  Data Type Conversion1/1 -> Out1/1
  Data Type Conversion/1 -> Data Type Conversion1/1, Display1/1, PWM/1

== system Semi_Final_integration/Subsystem9 ==
  In1 : Inport
  Derivative2 : Derivative
  Gain1 : Gain  Gain=KI
  Gain2 : Gain  Gain=KP
  Gain3 : Gain  Gain=KD
  Integrator2 : Integrator
  Subtract2 : Sum  Inputs=+++
  Out1 : Outport
  wires:
  Gain1/1 -> Integrator2/1
  Gain2/1 -> Subtract2/2
  Integrator2/1 -> Subtract2/1
  In1/1 -> Gain2/1, Gain3/1, Gain1/1
  Derivative2/1 -> Subtract2/3
  Gain3/1 -> Derivative2/1
  Subtract2/1 -> Out1/1

== system Semi_Final_integration/light_Ctrl ==
  light1 : Inport
  In2 : Inport  Port=2
  Drive_mode1 : Inport  Port=3
  Display1 : Display
  If : If  IfExpression=u1 == 0  ShowElse=off
  If Action Subsystem : Subsystem  TreatAsAtomicUnit=on
  Rate Transition : RateTransition  Integrity=off
  Rate Transition1 : RateTransition  Integrity=off  OutPortSampleTime=0.2
  Subsystem : Subsystem
  light_mode : Outport
  wires:
  If Action Subsystem/1(Out1) -> Rate Transition/1, Display1/1
  In2/1 -> Rate Transition1/1
  Rate Transition/1 -> Subsystem/2(sw3)
  Drive_mode1/1 -> If Action Subsystem/1(Drive_mode1)
  light1/1 -> Subsystem/1(light1)
  Subsystem/1(light_mode) -> light_mode/1
  If/1 -> If Action Subsystem/Action
  Rate Transition1/1 -> If/1

== system Semi_Final_integration/LED_B Ctrl/If Action Subsystem1 ==
  Input : Inport
  Action Port : ActionPort  ActionPortLabel=if(u1 ==1)
  Out1 : Outport
  wires:
  Input/1 -> Out1/1

== system Semi_Final_integration/LED_B Ctrl/If Action Subsystem3 ==
  Input : Inport
  Action Port : ActionPort  ActionPortLabel=else
  Out1 : Outport
  wires:
  Input/1 -> Out1/1

== system Semi_Final_integration/LED_R Ctrl/If Action Subsystem1 ==
  Action Port : ActionPort  ActionPortLabel=if(u1 ==1)
  Constant : Constant
  Out1 : Outport
  wires:
  Constant/1 -> Out1/1

== system Semi_Final_integration/LED_R Ctrl/If Action Subsystem3 ==
  Action Port : ActionPort  ActionPortLabel=else
  Constant : Constant  Value=0
  Out1 : Outport
  wires:
  Constant/1 -> Out1/1

== system Semi_Final_integration/State_Ctrl/ADAS_state ==
  In1 : Inport
  In2 : Inport  Port=2
  If : If  IfExpression=u1 == 0  ShowElse=off
  If Action Subsystem : Subsystem  TreatAsAtomicUnit=on
  If Action Subsystem1 : Subsystem  TreatAsAtomicUnit=on
  Rate Transition : RateTransition  Integrity=off
  Rate Transition2 : RateTransition  Integrity=off  OutPortSampleTime=0.2
  ADAS_state : Outport
  wires:
  In1/1 -> If Action Subsystem/Action
  If Action Subsystem/1(ADAS_state) -> ADAS_state/1
  In2/1 -> Rate Transition2/1
  Rate Transition2/1 -> If/1
  If/1 -> If Action Subsystem1/Action
  If Action Subsystem1/1(sw2) -> Rate Transition/1
  Rate Transition/1 -> If Action Subsystem/1(sw2)

== system Semi_Final_integration/State_Ctrl/drive_mode ==
  light_mode : Inport
  sw1 : Inport  Port=2
  A_state : Inport  Port=3
  Rate Transition : RateTransition  Integrity=off  OutPortSampleTime=0.01
  Rate Transition1 : RateTransition  Integrity=off
  Rate Transition2 : RateTransition  Integrity=off
  SW1 : Subsystem
  D_mode : Outport
  wires:
  SW1/1(Output) -> Rate Transition/1
  sw1/1 -> SW1/Trigger
  Rate Transition/1 -> D_mode/1
  light_mode/1 -> Rate Transition1/1
  A_state/1 -> Rate Transition2/1
  Rate Transition1/1 -> SW1/1(light_mode)
  Rate Transition2/1 -> SW1/2(A_state)

== system Semi_Final_integration/Subsystem2/Subsystem1 ==
  Data Type Conversion1 : DataTypeConversion  OutDataTypeStr=int32  SaturateOnIntegerOverflow=off  RndMeth=Floor
  Discrete Transfer Fcn : DiscreteTransferFcn  Numerator=num_Gd  Denominator=den_Gd
  Discrete Derivative : simulink/Discrete/Discrete Derivative  gainval=1.0  ICPrevScaledInput=0.0  OutMin=[]  OutMax=[]  OutDataType=fixdt(1, 16)  OutScaling=2^-10  DoSatur=off
  Display : Display
  Encoder : arduinosensorlib/Encoder  InputA=18  InputB=19  Mode=No reset  SampleTime=-1
  Gain1 : Gain  Gain=encoder_scale
  Gain2 : Gain  Gain=60/(2*pi)
  Out1 : Outport
  Out2 : Outport  Port=2
  wires:
  Gain1/1 -> Display/1, Gain2/1, Data Type Conversion1/1
  Encoder/1 -> Discrete Derivative/1
  Gain2/1 -> Out2/1
  Data Type Conversion1/1 -> Discrete Transfer Fcn/1
  Discrete Derivative/1 -> Gain1/1
  Discrete Transfer Fcn/1 -> Out1/1

== system Semi_Final_integration/Subsystem2/Subsystem2 ==
  Data Type Conversion1 : DataTypeConversion  OutDataTypeStr=int32  SaturateOnIntegerOverflow=off  RndMeth=Floor
  Discrete Transfer Fcn : DiscreteTransferFcn  Numerator=num_Gd  Denominator=den_Gd
  Discrete Derivative : simulink/Discrete/Discrete Derivative  gainval=1.0  ICPrevScaledInput=0.0  OutMin=[]  OutMax=[]  OutDataType=fixdt(1, 16)  OutScaling=2^-10  DoSatur=off
  Display : Display
  Encoder : arduinosensorlib/Encoder  InputA=18  InputB=19  Mode=No reset  SampleTime=-1
  Gain1 : Gain  Gain=encoder_scale
  Gain2 : Gain  Gain=60/(2*pi)
  Out1 : Outport
  Out2 : Outport  Port=2
  wires:
  Gain1/1 -> Display/1, Gain2/1, Data Type Conversion1/1
  Encoder/1 -> Discrete Derivative/1
  Gain2/1 -> Out2/1
  Data Type Conversion1/1 -> Discrete Transfer Fcn/1
  Discrete Derivative/1 -> Gain1/1
  Discrete Transfer Fcn/1 -> Out1/1

== system Semi_Final_integration/Subsystem2/Subsystem4 ==
  In1 : Inport
  Add : Sum  Inputs=+-
  Add1 : Sum
  Gain : Gain  Gain=Kb
  Transfer Fcn : TransferFcn  Numerator=Km  Denominator=[L R]
  Transfer Fcn1 : TransferFcn  Numerator=1  Denominator=[J Kf]
  Out1 : Outport
  wires:
  In1/1 -> Add/1
  ? -> Add1/1
  Add/1 -> Transfer Fcn/1
  Add1/1 -> Transfer Fcn1/1
  Transfer Fcn/1 -> Add1/2
  Gain/1 -> Add/2
  Transfer Fcn1/1 -> Gain/1, Out1/1

== system Semi_Final_integration/Subsystem2/Subsystem5 ==
  In1 : Inport
  Derivative1 : Derivative
  Gain4 : Gain  Gain=KI
  Gain5 : Gain  Gain=KP
  Gain6 : Gain  Gain=KD
  Integrator1 : Integrator
  Subtract1 : Sum  Inputs=+++
  Out1 : Outport
  wires:
  Subtract1/1 -> Out1/1
  In1/1 -> Gain5/1, Gain6/1, Gain4/1
  Integrator1/1 -> Subtract1/1
  Derivative1/1 -> Subtract1/3
  Gain6/1 -> Derivative1/1
  Gain5/1 -> Subtract1/2
  Gain4/1 -> Integrator1/1

== system Semi_Final_integration/Subsystem3/If Action Subsystem ==
  Action Port : ActionPort  ActionPortLabel=if(u1 == 1)
  Pulse Generator : DiscretePulseGenerator  PulseType=Time based  Period=0.2  PulseWidth=50
  Output : Outport
  wires:
  Pulse Generator/1 -> Output/1

== system Semi_Final_integration/Subsystem3/If Action Subsystem1 ==
  Action Port : ActionPort  ActionPortLabel=else
  Constant : Constant  Value=0
  Out1 : Outport
  wires:
  Constant/1 -> Out1/1

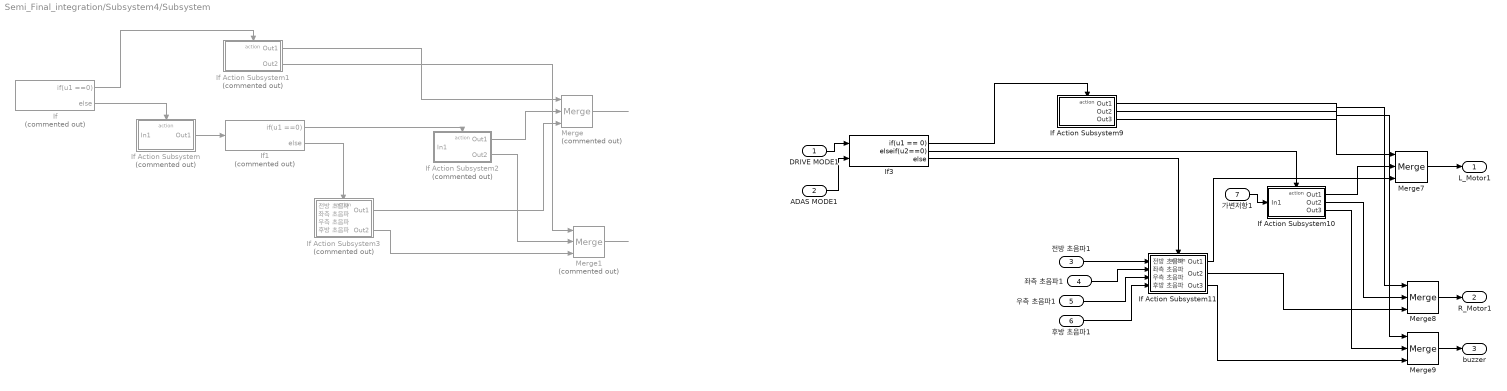
== system Semi_Final_integration/Subsystem4/Subsystem ==
  DRIVE MODE1 : Inport
  ADAS MODE1 : Inport  Port=2
  전방 초음파1 : Inport  Port=3
  좌측 초음파1 : Inport  Port=4
  우측 초음파1 : Inport  Port=5
  후방 초음파1 : Inport  Port=6
  가변저항1 : Inport  Port=7
  If : If  Commented=on  IfExpression=u1 ==0
  If Action Subsystem : Subsystem  Commented=on  TreatAsAtomicUnit=on
  If Action Subsystem1 : Subsystem  Commented=on  TreatAsAtomicUnit=on
  If Action Subsystem10 : Subsystem  TreatAsAtomicUnit=on
  If Action Subsystem11 : Subsystem  TreatAsAtomicUnit=on
  If Action Subsystem2 : Subsystem  Commented=on  TreatAsAtomicUnit=on
  If Action Subsystem3 : Subsystem  Commented=on  TreatAsAtomicUnit=on
  If Action Subsystem9 : Subsystem  TreatAsAtomicUnit=on
  If1 : If  Commented=on  IfExpression=u1 ==0
  If3 : If  NumInputs=2  IfExpression=u1 == 0  ElseIfExpressions=u2==0
  Merge : Merge  Commented=on  Inputs=3
  Merge1 : Merge  Commented=on  Inputs=3
  Merge7 : Merge  Inputs=3
  Merge8 : Merge  Inputs=3
  Merge9 : Merge  Inputs=3
  L_Motor1 : Outport
  R_Motor1 : Outport  Port=2
  buzzer : Outport  Port=3
  wires:
  If/2 -> If Action Subsystem/Action
  If/1 -> If Action Subsystem1/Action
  ? -> If Action Subsystem/1(In1)
  If Action Subsystem/1(Out1) -> If1/1
  If1/1 -> If Action Subsystem2/Action
  ? -> If Action Subsystem2/1(In1)
  If1/2 -> If Action Subsystem3/Action
  If Action Subsystem1/1(Out1) -> Merge/1
  If Action Subsystem2/1(Out1) -> Merge/2
  If Action Subsystem3/1(Out1) -> Merge/3
  If Action Subsystem1/2(Out2) -> Merge1/1
  If Action Subsystem2/2(Out2) -> Merge1/2
  If Action Subsystem3/2(Out2) -> Merge1/3
  Merge/1 -> ?
  Merge1/1 -> ?
  ? -> If Action Subsystem3/1(전방 초음파)
  ? -> If Action Subsystem3/2(좌측 초음파)
  ? -> If Action Subsystem3/3(우측 초음파)
  ? -> If Action Subsystem3/4(후방 초음파)
  후방 초음파1/1 -> If Action Subsystem11/4(후방 초음파)
  Merge9/1 -> buzzer/1
  우측 초음파1/1 -> If Action Subsystem11/3(우측 초음파)
  If Action Subsystem11/1(Out1) -> Merge7/3
  Merge8/1 -> R_Motor1/1
  If Action Subsystem9/2(Out2) -> Merge8/1
  If3/3 -> If Action Subsystem11/Action
  If Action Subsystem10/1(Out1) -> Merge7/2
  Merge7/1 -> L_Motor1/1
  If3/1 -> If Action Subsystem9/Action
  If Action Subsystem9/1(Out1) -> Merge7/1
  If Action Subsystem9/3(Out3) -> Merge9/1
  좌측 초음파1/1 -> If Action Subsystem11/2(좌측 초음파)
  If Action Subsystem11/3(Out3) -> Merge9/3
  전방 초음파1/1 -> If Action Subsystem11/1(전방 초음파)
  If Action Subsystem10/2(Out2) -> Merge8/2
  If Action Subsystem10/3(Out3) -> Merge9/2
  If3/2 -> If Action Subsystem10/Action
  If Action Subsystem11/2(Out2) -> Merge8/3
  DRIVE MODE1/1 -> If3/1
  가변저항1/1 -> If Action Subsystem10/1(In1)
  ADAS MODE1/1 -> If3/2

== system Semi_Final_integration/light_Ctrl/If Action Subsystem ==
  Drive_mode1 : Inport
  Action Port : ActionPort  ActionPortLabel=if(u1 == 0)
  Constant : Constant
  Constant1 : Constant  Value=3
  Constant2 : Constant  Value=0
  Delay : Delay  DelayLength=1
  If : If  IfExpression=u1 == 1
  If Action Subsystem : Subsystem  TreatAsAtomicUnit=on
  If Action Subsystem1 : Subsystem  TreatAsAtomicUnit=on
  Merge : Merge
  Mod : Math  Operator=mod
  Plus : Sum
  Out1 : Outport
  wires:
  Mod/1 -> Out1/1, Delay/1
  Delay/1 -> Plus/2
  Plus/1 -> Mod/1
  Constant1/1 -> Mod/2
  If/1 -> If Action Subsystem/Action
  If/2 -> If Action Subsystem1/Action
  Constant/1 -> If Action Subsystem/1(In1)
  Constant2/1 -> If Action Subsystem1/1(In1)
  If Action Subsystem/1(Out1) -> Merge/1
  If Action Subsystem1/1(Out1) -> Merge/2
  Merge/1 -> Plus/1
  Drive_mode1/1 -> If/1

== system Semi_Final_integration/light_Ctrl/Subsystem ==
  light1 : Inport
  sw3 : Inport  Port=2
  Chart1 : Stateflow chart  Commented=on  TreatAsAtomicUnit=on
  Subsystem : Subsystem
  light_mode : Outport
  wires:
  light1/1 -> Subsystem/1(light)
  sw3/1 -> light_mode/1, Subsystem/2(light_mode)

== system Semi_Final_integration/State_Ctrl/ADAS_state/If Action Subsystem ==
  sw2 : Inport
  Action Port : ActionPort  ActionPortLabel=if(u1 ==1)
  ADAS_state : Outport
  wires:
  sw2/1 -> ADAS_state/1

== system Semi_Final_integration/State_Ctrl/ADAS_state/If Action Subsystem1 ==
  Action Port : ActionPort  ActionPortLabel=if(u1 == 0)
  Constant2 : Constant
  Constant3 : Constant  Value=2
  Delay1 : Delay  DelayLength=1  InitialCondition=0
  Mod1 : Math  Operator=mod
  Sum : Sum  Inputs=|++
  sw2 : Outport
  wires:
  Mod1/1 -> sw2/1
  Delay1/1 -> Sum/2
  Constant3/1 -> Mod1/2
  Sum/1 -> Delay1/1, Mod1/1
  Constant2/1 -> Sum/1

== system Semi_Final_integration/State_Ctrl/drive_mode/SW1 ==
  light_mode : Inport
  A_state : Inport  Port=2
  function : TriggerPort  TriggerType=function-call  VariantControl=(inherit)
  Constant2 : Constant
  Delay : Delay  DelayLength=1
  If : If  IfExpression=u1 == 0  ElseIfExpressions=u1 == 1  ShowElse=off
  If Action Subsystem : Subsystem  TreatAsAtomicUnit=on
  If Action Subsystem1 : Subsystem  TreatAsAtomicUnit=on
  Merge : Merge
  Output : Outport
  wires:
  Delay/1 -> If/1
  If/1 -> If Action Subsystem/Action
  Constant2/1 -> If Action Subsystem/1(In1)
  If/2 -> If Action Subsystem1/Action
  If Action Subsystem/1(Out1) -> Merge/1
  light_mode/1 -> If Action Subsystem1/1(light_mode)
  A_state/1 -> If Action Subsystem1/2(A_state)
  If Action Subsystem1/1(Out1) -> Merge/2
  Merge/1 -> Delay/1, Output/1

== system Semi_Final_integration/Subsystem4/Subsystem/If Action Subsystem ==
  In1 : Inport
  Action Port : ActionPort
  Out1 : Outport
  wires:
  In1/1 -> Out1/1

== system Semi_Final_integration/Subsystem4/Subsystem/If Action Subsystem1 ==
  Action Port : ActionPort
  Constant : Constant  Value=0
  Constant1 : Constant  Value=0
  Out1 : Outport
  Out2 : Outport  Port=2
  wires:
  Constant/1 -> Out1/1
  Constant1/1 -> Out2/1
